simulink model "PMSM_Simulink"  (R2024b)
settings: Solver=ode45  StartTime=0.0  StopTime=10.0  MaxStep=1e-3  RelTol=1e-6  AbsTol=1e-8
values from neighbouring files (symbols this model uses):
  B = 0.08    [PMSM_main_code.m]
  isd0 = cosd(Beta_fixed)*Imag0    [PMSM_main_code.m]
  isq0 = sind(Beta_fixed)*Imag0    [PMSM_main_code.m]
  J = 0.0125    [PMSM_main_code.m]
  Lsd = Laa0+Lab0+3/2*Laa2    (= 0.0345)    [PMSM_main_code.m]
  Lsq = Laa0+Lab0-3/2*Laa2    (= 0.0855)    [PMSM_main_code.m]
  np = 2    [PMSM_main_code.m]
  Psim = 0.822    [PMSM_main_code.m]
  Rs = 1.33    [PMSM_main_code.m]
  theta0 = 0    [PMSM_main_code.m]
  TL_extra = 12    [PMSM_main_code.m]
  TL_extra_time = 0.5    [PMSM_main_code.m]
  usd0 = Rs*isd0-ws*Lsq*isq0    [PMSM_main_code.m]
  usq0 = Rs*isq0+ws*Lsd*isd0+ws*Psim    [PMSM_main_code.m]
  wr0 = ws    (= 314.159265359)    [PMSM_main_code.m]
  ws = 2*pi*fs    (= 314.159265359)    [PMSM_main_code.m]
undefined symbols (not defined in the file or in its folder): j
settings Model: Creator=e6zebra  LastModifiedBy=Admin
settings SolverCC: AutoScaleAbsTol=off  AlgebraicLoopSolver=TrustRegion
settings DataIOCC: SaveFormat=Array  SignalLoggingSaveFormat=ModelDataLogs  ReturnWorkspaceOutputs=off
settings OptimizationCC: BlockReduction=off  BooleanDataType=off  ExpressionDepthLimit=2147483647  InitFltsAndDblsToZero=on  LifeSpan=inf
settings DebuggingCC: SaveWithParameterizedLinksMsg=none  UnderspecifiedInitializationDetection=Classic  MergeDetectMultiDrivingBlocksExec=none  SignalResolutionControl=TryResolveAllWithWarning  MultiTaskDSMMsg=warning  MultiTaskCondExecSysMsg=none  FcnCallInpInsideContextMsg=warning  UnconnectedInputMsg=warning  UnconnectedOutputMsg=warning  UnconnectedLineMsg=warning  StateNameClashWarn=warning  SFUnexpectedBacktrackingDiag=warning  SFNoUnconditionalDefaultTransitionDiag=warning  SFExecutionAtInitializationDiag=none  ArithmeticOperatorsInVariantConditions=warning
settings HardwareCC: ProdBitPerPointer=32  ProdBitPerSizeT=32  ProdBitPerPtrDiffT=32  ProdLargestAtomicFloat=None  ProdIntDivRoundTo=Undefined  ProdEndianess=Unspecified  ProdWordSize=32  ProdHWDeviceType=32-bit Generic  TargetUnknown=on
settings ModelReferenceCC: EnableRefExpFcnMdlSchedulingChecks=on  PropagateSignalLabelsOutOfModel=off
settings SFSimCC: SimUseLocalCustomCode=off  CustomCodeUndefinedFunction=UseInterfaceOnly
settings RTWCC: TemplateMakefile=grt.tmf  RTWUseLocalCustomCode=off  GPUComputeCapability=3.5
settings CodeAppCC: StateflowObjectComments=on
settings GRTTargetCC: TargetFcnLib=ansi_tfl_tmw.mat  TargetLangStandard=C89/C90 (ANSI)  CombineOutputUpdateFcns=off  GRTInterface=on
settings ConfigComp: CovMetricSettings=dw  CovSaveCumulativeToWorkspaceVar=on  CovSaveSingleToWorkspaceVar=on  CovExternalEMLEnable=off

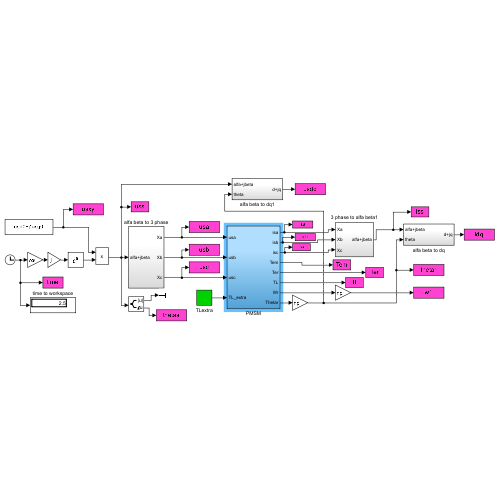
[thumbnail: Simulink's stored preview of the top-level diagram]
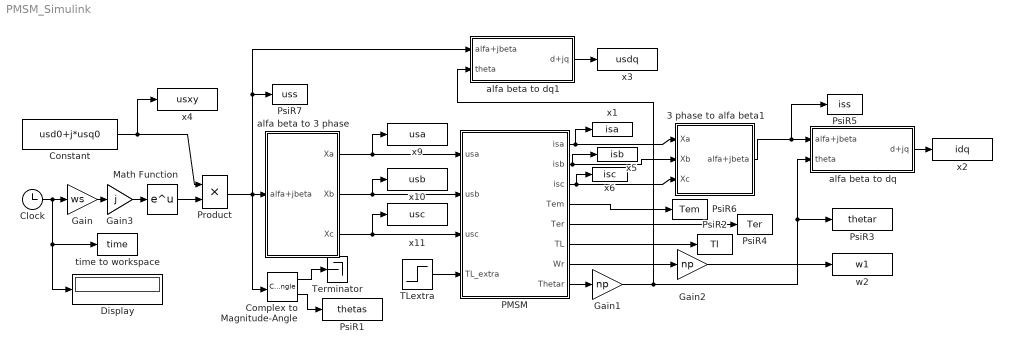
== system PMSM_Simulink ==
  3 phase to alfa beta1 : Subsystem
  Clock : Clock
  Complex to Magnitude-Angle : ComplexToMagnitudeAngle
  Constant : Constant  Value=usd0+j*usq0
  Display : Display
  Gain : Gain  Gain=ws
  Gain1 : Gain  Gain=np
  Gain2 : Gain  Gain=np
  Gain3 : Gain  Gain=j  SaturateOnIntegerOverflow=on  OutDataTypeStr=Inherit: Same as input  ParamDataTypeStr=Inherit: Same as input
  Math Function : Math  SignedPower=on
  PMSM : Subsystem
  Product : Product  SaturateOnIntegerOverflow=on  OutDataTypeStr=Inherit: Same as first input
  PsiR1 : ToWorkspace  VariableName=thetas  SampleTime=-1
  PsiR2 : ToWorkspace  VariableName=Tl  SampleTime=-1
  PsiR3 : ToWorkspace  VariableName=thetar  SampleTime=-1
  PsiR4 : ToWorkspace  VariableName=Ter  SampleTime=-1
  PsiR5 : ToWorkspace  VariableName=iss  SampleTime=-1
  PsiR6 : ToWorkspace  VariableName=Tem  SampleTime=-1
  PsiR7 : ToWorkspace  VariableName=uss  SampleTime=-1
  TLextra : Step  Time=TL_extra_time  After=TL_extra  SampleTime=0
  Terminator : Terminator
  alfa beta to 3 phase : Subsystem
  alfa beta to dq : Subsystem
  alfa beta to dq1 : Subsystem
  time to workspace : ToWorkspace  VariableName=time  SampleTime=-1
  w2 : ToWorkspace  VariableName=w1  SampleTime=-1
  x1 : ToWorkspace  VariableName=isa  SampleTime=-1
  x10 : ToWorkspace  VariableName=usb  SampleTime=-1
  x11 : ToWorkspace  VariableName=usc  SampleTime=-1
  x2 : ToWorkspace  VariableName=idq  SampleTime=-1
  x3 : ToWorkspace  VariableName=usdq  SampleTime=-1
  x4 : ToWorkspace  VariableName=usxy  SampleTime=-1
  x5 : ToWorkspace  VariableName=isb  SampleTime=-1
  x6 : ToWorkspace  VariableName=isc  SampleTime=-1
  x9 : ToWorkspace  VariableName=usa  SampleTime=-1
  wires:
  Clock/1 -> Gain/1, time to workspace/1, Display/1
  PMSM/7(Wr) -> Gain2/1
  alfa beta to dq/1(d+jq) -> x2/1
  TLextra/1 -> PMSM/4(TL_extra)
  Gain/1 -> Gain3/1
  Constant/1 -> x4/1, Product/1
  PMSM/8(Thetar) -> Gain1/1
  PMSM/6(TL) -> PsiR2/1
  PMSM/5(Ter) -> PsiR4/1
  alfa beta to dq1/1(d+jq) -> x3/1
  Gain1/1 -> alfa beta to dq1/2(theta), alfa beta to dq/2(theta), PsiR3/1
  Gain2/1 -> w2/1
  PMSM/3(isc) -> x6/1, 3 phase to alfa beta1/3(Xc)
  PMSM/2(isb) -> x5/1, 3 phase to alfa beta1/2(Xb)
  PMSM/1(isa) -> 3 phase to alfa beta1/1(Xa), x1/1
  3 phase to alfa beta1/1(alfa+jbeta) -> PsiR5/1, alfa beta to dq/1(alfa+jbeta)
  alfa beta to 3 phase/1(Xa) -> PMSM/1(usa), x9/1
  alfa beta to 3 phase/2(Xb) -> PMSM/2(usb), x10/1
  alfa beta to 3 phase/3(Xc) -> PMSM/3(usc), x11/1
  Gain3/1 -> Math Function/1
  Math Function/1 -> Product/2
  Complex to Magnitude-Angle/2 -> PsiR1/1
  Complex to Magnitude-Angle/1 -> Terminator/1
  Product/1 -> alfa beta to 3 phase/1(alfa+jbeta), alfa beta to dq1/1(alfa+jbeta), PsiR7/1, Complex to Magnitude-Angle/1
  PMSM/4(Tem) -> PsiR6/1

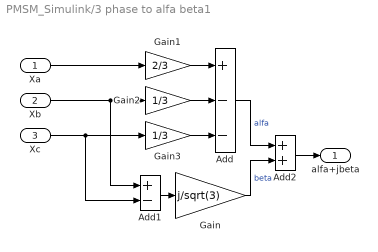
== system PMSM_Simulink/3 phase to alfa beta1 ==
  Xa : Inport
  Xb : Inport  Port=2
  Xc : Inport  Port=3
  Add : Sum  Inputs=+--
  Add1 : Sum  Inputs=+-
  Add2 : Sum
  Gain : Gain  Gain=j/sqrt(3)
  Gain1 : Gain  Gain=2/3
  Gain2 : Gain  Gain=1/3
  Gain3 : Gain  Gain=1/3
  alfa+jbeta : Outport  VectorParamsAs1DForOutWhenUnconnected=off
  wires:
  Add1/1 -> Gain/1
  Add2/1 -> alfa+jbeta/1
  Gain/1 -> Add2/2  "beta"
  Add/1 -> Add2/1  "alfa"
  Gain3/1 -> Add/3
  Gain2/1 -> Add/2
  Gain1/1 -> Add/1
  Xa/1 -> Gain1/1
  Xb/1 -> Gain2/1, Add1/1
  Xc/1 -> Gain3/1, Add1/2

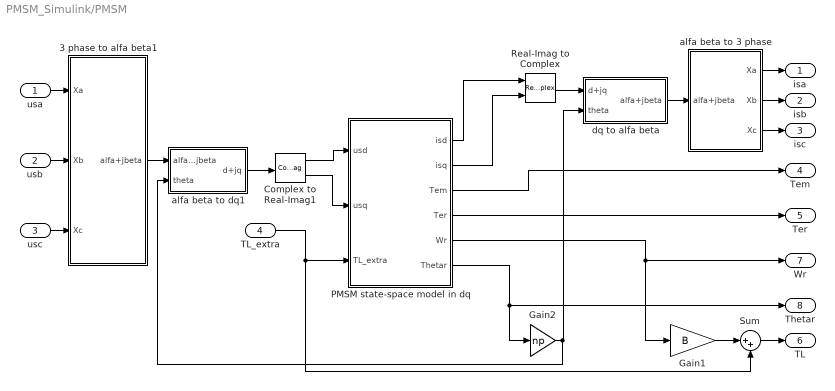
== system PMSM_Simulink/PMSM ==
  usa : Inport
  usb : Inport  Port=2
  usc : Inport  Port=3
  TL_extra : Inport  Port=4
  3 phase to alfa beta1 : Subsystem
  Complex to Real-Imag1 : ComplexToRealImag
  Gain1 : Gain  Gain=B
  Gain2 : Gain  Gain=np
  PMSM state-space model in dq : Subsystem
  Real-Imag to Complex : RealImagToComplex
  Sum : Sum  Inputs=|++  SaturateOnIntegerOverflow=on
  alfa beta to 3 phase : Subsystem
  alfa beta to dq1 : Subsystem
  dq to alfa beta : Subsystem
  isa : Outport  VectorParamsAs1DForOutWhenUnconnected=off
  isb : Outport  Port=2  VectorParamsAs1DForOutWhenUnconnected=off
  isc : Outport  Port=3  VectorParamsAs1DForOutWhenUnconnected=off
  Tem : Outport  Port=4  VectorParamsAs1DForOutWhenUnconnected=off
  Ter : Outport  Port=5  VectorParamsAs1DForOutWhenUnconnected=off
  TL : Outport  Port=6  VectorParamsAs1DForOutWhenUnconnected=off
  Wr : Outport  Port=7  VectorParamsAs1DForOutWhenUnconnected=off
  Thetar : Outport  Port=8  VectorParamsAs1DForOutWhenUnconnected=off
  wires:
  TL_extra/1 -> Sum/2, PMSM state-space model in dq/3(TL_extra)
  Gain1/1 -> Sum/1
  Sum/1 -> TL/1
  usc/1 -> 3 phase to alfa beta1/3(Xc)
  usb/1 -> 3 phase to alfa beta1/2(Xb)
  usa/1 -> 3 phase to alfa beta1/1(Xa)
  alfa beta to 3 phase/1(Xa) -> isa/1
  alfa beta to 3 phase/3(Xc) -> isc/1
  alfa beta to 3 phase/2(Xb) -> isb/1
  Real-Imag to Complex/1 -> dq to alfa beta/1(d+jq)
  dq to alfa beta/1(alfa+jbeta) -> alfa beta to 3 phase/1(alfa+jbeta)
  3 phase to alfa beta1/1(alfa+jbeta) -> alfa beta to dq1/1(alfa+jbeta)
  Gain2/1 -> alfa beta to dq1/2(theta), dq to alfa beta/2(theta)
  alfa beta to dq1/1(d+jq) -> Complex to Real-Imag1/1
  PMSM state-space model in dq/5(Wr) -> Gain1/1, Wr/1
  PMSM state-space model in dq/6(Thetar) -> Gain2/1, Thetar/1
  Complex to Real-Imag1/1 -> PMSM state-space model in dq/1(usd)
  Complex to Real-Imag1/2 -> PMSM state-space model in dq/2(usq)
  PMSM state-space model in dq/1(isd) -> Real-Imag to Complex/1
  PMSM state-space model in dq/2(isq) -> Real-Imag to Complex/2
  PMSM state-space model in dq/3(Tem) -> Tem/1
  PMSM state-space model in dq/4(Ter) -> Ter/1

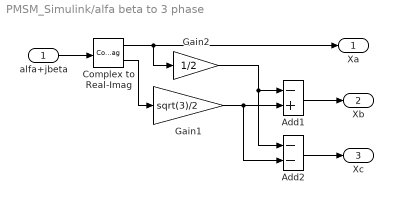
== system PMSM_Simulink/alfa beta to 3 phase ==
  alfa+jbeta : Inport
  Add1 : Sum  Inputs=-+
  Add2 : Sum  Inputs=--
  Complex to Real-Imag : ComplexToRealImag
  Gain1 : Gain  Gain=sqrt(3)/2
  Gain2 : Gain  Gain=1/2
  Xa : Outport  VectorParamsAs1DForOutWhenUnconnected=off
  Xb : Outport  Port=2  VectorParamsAs1DForOutWhenUnconnected=off
  Xc : Outport  Port=3  VectorParamsAs1DForOutWhenUnconnected=off
  wires:
  alfa+jbeta/1 -> Complex to Real-Imag/1
  Complex to Real-Imag/1 -> Xa/1, Gain2/1
  Add2/1 -> Xc/1
  Add1/1 -> Xb/1
  Complex to Real-Imag/2 -> Gain1/1
  Gain1/1 -> Add1/2, Add2/2
  Gain2/1 -> Add1/1, Add2/1

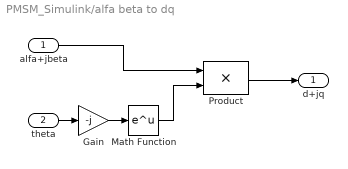
== system PMSM_Simulink/alfa beta to dq ==
  alfa+jbeta : Inport
  theta : Inport  Port=2
  Gain : Gain  Gain=-j  SaturateOnIntegerOverflow=on  OutDataTypeStr=Inherit: Same as input  ParamDataTypeStr=Inherit: Same as input
  Math Function : Math  SignedPower=on
  Product : Product  SaturateOnIntegerOverflow=on  OutDataTypeStr=Inherit: Same as first input
  d+jq : Outport  VectorParamsAs1DForOutWhenUnconnected=off
  wires:
  theta/1 -> Gain/1
  Gain/1 -> Math Function/1
  Math Function/1 -> Product/2
  alfa+jbeta/1 -> Product/1
  Product/1 -> d+jq/1

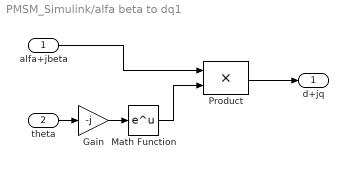
== system PMSM_Simulink/alfa beta to dq1 ==
  alfa+jbeta : Inport
  theta : Inport  Port=2
  Gain : Gain  Gain=-j  SaturateOnIntegerOverflow=on  OutDataTypeStr=Inherit: Same as input  ParamDataTypeStr=Inherit: Same as input
  Math Function : Math  SignedPower=on
  Product : Product  SaturateOnIntegerOverflow=on  OutDataTypeStr=Inherit: Same as first input
  d+jq : Outport  VectorParamsAs1DForOutWhenUnconnected=off
  wires:
  theta/1 -> Gain/1
  Gain/1 -> Math Function/1
  Math Function/1 -> Product/2
  alfa+jbeta/1 -> Product/1
  Product/1 -> d+jq/1

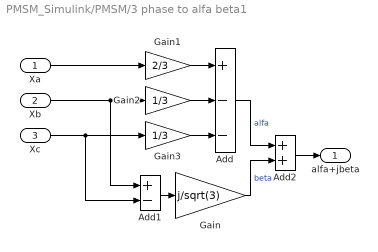
== system PMSM_Simulink/PMSM/3 phase to alfa beta1 ==
  Xa : Inport
  Xb : Inport  Port=2
  Xc : Inport  Port=3
  Add : Sum  Inputs=+--
  Add1 : Sum  Inputs=+-
  Add2 : Sum
  Gain : Gain  Gain=j/sqrt(3)
  Gain1 : Gain  Gain=2/3
  Gain2 : Gain  Gain=1/3
  Gain3 : Gain  Gain=1/3
  alfa+jbeta : Outport  VectorParamsAs1DForOutWhenUnconnected=off
  wires:
  Add1/1 -> Gain/1
  Add2/1 -> alfa+jbeta/1
  Gain/1 -> Add2/2  "beta"
  Add/1 -> Add2/1  "alfa"
  Gain3/1 -> Add/3
  Gain2/1 -> Add/2
  Gain1/1 -> Add/1
  Xa/1 -> Gain1/1
  Xb/1 -> Gain2/1, Add1/1
  Xc/1 -> Gain3/1, Add1/2

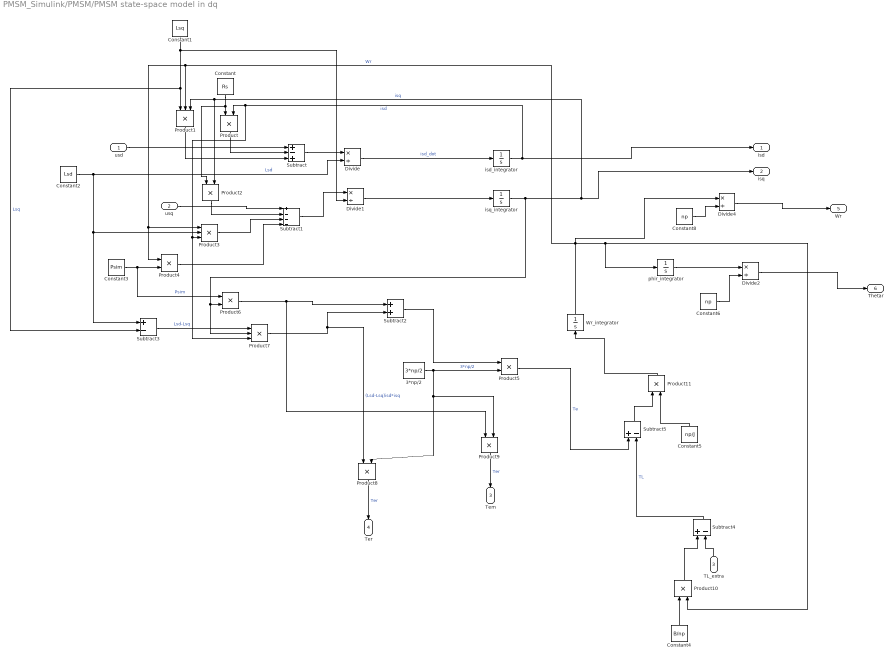
== system PMSM_Simulink/PMSM/PMSM state-space model in dq ==
  usd : Inport
  usq : Inport  Port=2
  TL_extra : Inport  Port=3
  3*np/2 : Constant  Value=3*np/2
  Constant : Constant  Value=Rs
  Constant1 : Constant  Value=Lsq
  Constant2 : Constant  Value=Lsd
  Constant3 : Constant  Value=Psim
  Constant4 : Constant  Value=B/np
  Constant5 : Constant  Value=np/J
  Constant6 : Constant  Value=np
  Constant8 : Constant  Value=np
  Divide{,1..2,4} (4 alike) : Product  Inputs=*/
  Product{,2,4..6,8..11} (9 alike) : Product
  Product1 : Product  Inputs=3
  Product3 : Product  Inputs=3
  Product7 : Product  Inputs=3
  Subtract : Sum  Inputs=+-+
  Subtract1 : Sum  Inputs=+---
  Subtract2 : Sum
  Subtract3 : Sum  Inputs=+-
  Subtract4 : Sum  Inputs=+-
  Subtract5 : Sum  Inputs=+-
  Wr_integrator : Integrator  InitialCondition=wr0
  isd_integrator : Integrator  InitialCondition=isd0
  isq_integrator : Integrator  InitialCondition=isq0
  phir_integrator : Integrator  InitialCondition=theta0
  isd : Outport  VectorParamsAs1DForOutWhenUnconnected=off
  isq : Outport  Port=2  VectorParamsAs1DForOutWhenUnconnected=off
  Tem : Outport  Port=3  VectorParamsAs1DForOutWhenUnconnected=off
  Ter : Outport  Port=4  VectorParamsAs1DForOutWhenUnconnected=off
  Wr : Outport  Port=5  VectorParamsAs1DForOutWhenUnconnected=off
  Thetar : Outport  Port=6  VectorParamsAs1DForOutWhenUnconnected=off
  wires:
  Product11/1 -> Wr_integrator/1
  Divide1/1 -> isq_integrator/1
  Divide/1 -> isd_integrator/1  "isd_dot"
  isd_integrator/1 -> isd/1, Product7/3, Product3/3, Product/2  "isd"
  usd/1 -> Subtract/1
  Constant/1 -> Product2/1, Product/1
  Product/1 -> Subtract/2
  Wr_integrator/1 -> Divide4/1, Product1/2, Product4/1, Product3/1, phir_integrator/1, Product10/2  "Wr"
  Constant1/1 -> Product1/1, Subtract3/2, Divide1/2  "Lsq"
  Product1/1 -> Subtract/3
  isq_integrator/1 -> Product7/2, Product6/2, Product1/3, Product2/2, isq/1  "isq"
  Subtract/1 -> Divide/1
  Constant2/1 -> Product3/2, Subtract3/1, Divide/2  "Lsd"
  usq/1 -> Subtract1/1
  Product2/1 -> Subtract1/2
  Product3/1 -> Subtract1/3
  Constant3/1 -> Product6/1, Product4/2  "Psim"
  Product4/1 -> Subtract1/4
  Subtract1/1 -> Divide1/1
  3*np/2/1 -> Product9/2, Product8/2, Product5/2  "3*np/2"
  Product6/1 -> Product9/1, Subtract2/1
  Subtract3/1 -> Product7/1  "Lsd-Lsq"
  Product7/1 -> Product8/1, Subtract2/2  "(Lsd-Lsq)isd*isq"
  Subtract2/1 -> Product5/1
  Product5/1 -> Subtract5/1  "Te"
  Product8/1 -> Ter/1  "Ter"
  Product9/1 -> Tem/1  "Ter"
  Constant4/1 -> Product10/1
  Product10/1 -> Subtract4/1
  TL_extra/1 -> Subtract4/2
  Subtract4/1 -> Subtract5/2  "TL"
  Subtract5/1 -> Product11/1
  Constant5/1 -> Product11/2
  phir_integrator/1 -> Divide2/1
  Constant6/1 -> Divide2/2
  Divide2/1 -> Thetar/1
  Constant8/1 -> Divide4/2
  Divide4/1 -> Wr/1

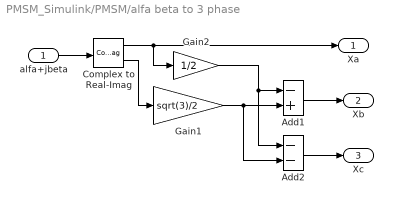
== system PMSM_Simulink/PMSM/alfa beta to 3 phase ==
  alfa+jbeta : Inport
  Add1 : Sum  Inputs=-+
  Add2 : Sum  Inputs=--
  Complex to Real-Imag : ComplexToRealImag
  Gain1 : Gain  Gain=sqrt(3)/2
  Gain2 : Gain  Gain=1/2
  Xa : Outport  VectorParamsAs1DForOutWhenUnconnected=off
  Xb : Outport  Port=2  VectorParamsAs1DForOutWhenUnconnected=off
  Xc : Outport  Port=3  VectorParamsAs1DForOutWhenUnconnected=off
  wires:
  alfa+jbeta/1 -> Complex to Real-Imag/1
  Complex to Real-Imag/1 -> Xa/1, Gain2/1
  Add2/1 -> Xc/1
  Add1/1 -> Xb/1
  Complex to Real-Imag/2 -> Gain1/1
  Gain1/1 -> Add1/2, Add2/2
  Gain2/1 -> Add1/1, Add2/1

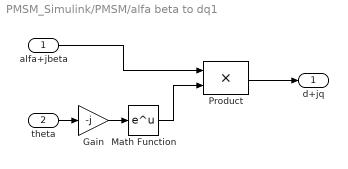
== system PMSM_Simulink/PMSM/alfa beta to dq1 ==
  alfa+jbeta : Inport
  theta : Inport  Port=2
  Gain : Gain  Gain=-j  SaturateOnIntegerOverflow=on  OutDataTypeStr=Inherit: Same as input  ParamDataTypeStr=Inherit: Same as input
  Math Function : Math  SignedPower=on
  Product : Product  SaturateOnIntegerOverflow=on  OutDataTypeStr=Inherit: Same as first input
  d+jq : Outport  VectorParamsAs1DForOutWhenUnconnected=off
  wires:
  theta/1 -> Gain/1
  Gain/1 -> Math Function/1
  Math Function/1 -> Product/2
  alfa+jbeta/1 -> Product/1
  Product/1 -> d+jq/1

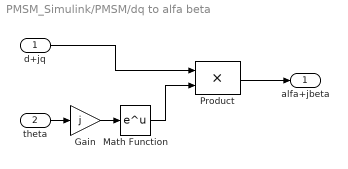
== system PMSM_Simulink/PMSM/dq to alfa beta ==
  d+jq : Inport
  theta : Inport  Port=2
  Gain : Gain  Gain=j  SaturateOnIntegerOverflow=on  OutDataTypeStr=Inherit: Same as input  ParamDataTypeStr=Inherit: Same as input
  Math Function : Math  SignedPower=on
  Product : Product  SaturateOnIntegerOverflow=on  OutDataTypeStr=Inherit: Same as first input
  alfa+jbeta : Outport  VectorParamsAs1DForOutWhenUnconnected=off
  wires:
  theta/1 -> Gain/1
  Gain/1 -> Math Function/1
  Math Function/1 -> Product/2
  d+jq/1 -> Product/1
  Product/1 -> alfa+jbeta/1
